simulink model "problem1"  (R2020a)
settings: Solver=VariableStepAuto  StartTime=0.0  StopTime=10.0  RelTol=1e-3
settings Model: Creator=Jake  LastModifiedBy=Jake

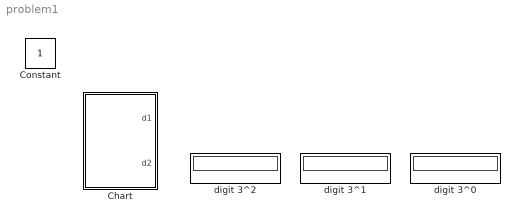
== system problem1 ==
  Chart : Stateflow chart  TreatAsAtomicUnit=on
  Constant : Constant
  digit 3^0 : Display
  digit 3^1 : Display
  digit 3^2 : Display
  wires:
  ? -> digit 3^0/1
  ? -> digit 3^2/1
  ? -> digit 3^1/1

== stateflow chart problem1/Chart ==
  state digit1 [parallel]
    settings: executionOrder=1
    state one
      en:
      d1=1;
    state two
      en:
      d1=2;
    state three
      en:
      d1=3;
    state zero
      en:
      d1=0;
    state four
      en:
      d1=4;
    digit1.three -> digit1.four : inputClick
    digit1.zero -> digit1.one : inputClick
    digit1.one -> digit1.two : inputClick
    digit1.two -> digit1.three : inputClick
    (default) -> digit1.zero
    digit1.four -> digit1.zero : inputClick/{digit2.inc2}
  state digit2 [parallel]
    settings: executionOrder=2
    state one
      en:
      d2=1;
    state two
      en:
      d2=2;
    state three
      en:
      d2=3;
    state four
      en:
      d2=4;
    state zero
      en:
      d2=0;
    digit2.three -> digit2.four : inc2
    digit2.one -> digit2.two : inc2
    digit2.two -> digit2.three : inc2
    digit2.zero -> digit2.one : inc2
    (default) -> digit2.zero
    digit2.four -> digit2.zero : inc2/{digit3.inc3}
  state digit3 [parallel]
    settings: executionOrder=3
    state one
      en:
      d3=1;
    state two
      en:
      d3=2;
    state three
      en:
      d2=3;
    state zero
      en:
      d3=0;
    state four
      en:
      d2=4;
    (default) -> digit3.zero
  data: d1 output; d2 output
  events: inc2 local FUNCTION_CALL_EVENT; inputClick local FUNCTION_CALL_EVENT
